simulink model "Testbed_OpenLoop"  (R2024b)
settings: Solver=VariableStepAuto  StartTime=0.0  StopTime=tf  RelTol=1e-3
values from neighbouring files (symbols this model uses):
  gamma1_initial = deg2rad(0)    [CMG_Testbed_Attitude_Control.m]
  gamma2_initial = deg2rad(0)    [CMG_Testbed_Attitude_Control.m]
libraries: simulink_extras x3, cstblocks x1
settings Model: Creator=lanhi  LastModifiedBy=lanhi

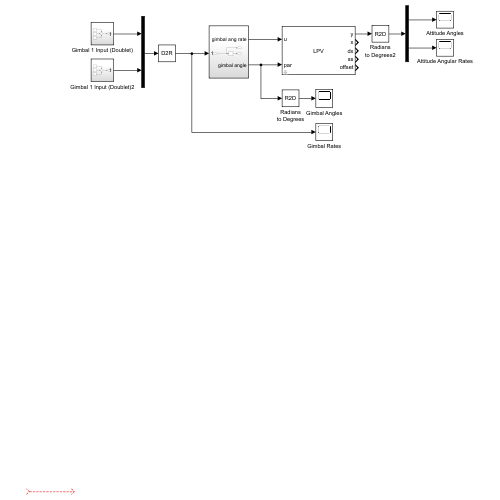
[thumbnail: Simulink's stored preview of the top-level diagram]
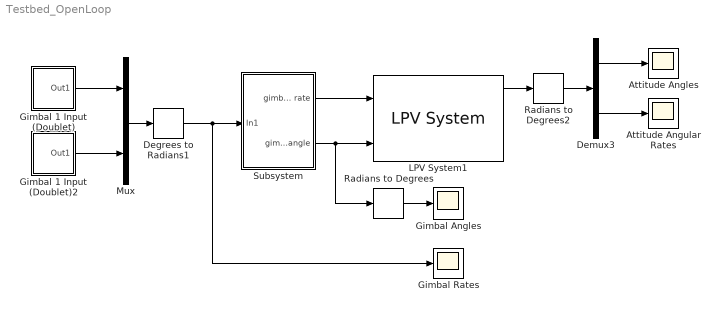
== system Testbed_OpenLoop ==
  Attitude Angles : Scope
  Attitude Angular Rates : Scope
  Degrees to Radians1 : simulink_extras/Transformations/Degrees to Radians
  Demux3 : Demux  Outputs=2
  Gimbal 1 Input (Doublet) : Subsystem
  Gimbal 1 Input (Doublet)2 : Subsystem
  Gimbal Angles : Scope
  Gimbal Rates : Scope
  LPV System1 : cstblocks/Linear Parameter Varying/LPV System  sys=ICs  InitialConditionSource=internal  InitialCondition=[deg2rad(0),0]  opSpecOption=Specify offsets as double arrays  uOffset=0  yOffset=0  xOffset=0  opEquilOption=on  dxOffset=0  AFixed=false  BFixed=false  CFixed=false  DFixed=false  uDelayFixed=false  yDelayFixed=false  iDelayFixed=false  sysFixedOption=First model in state-space array  sysFixed=[]  IMethod=Linear  EMethod=Clip  IndexSearch=Binary search  IndexBegin=on  OutputX=on  OutputXdot=on  OutputLTI=on  OutputOP=on  DataType=double  InitBufferSize=1024  FixedBuffer=off  SimMode=Interpreted execution  Offset=struct
  Mux : Mux  Inputs=2
  Radians to Degrees : simulink_extras/Transformations/Radians to Degrees
  Radians to Degrees2 : simulink_extras/Transformations/Radians to Degrees
  Subsystem : Subsystem
  wires:
  ? -> ?
  Radians to Degrees/1 -> Gimbal Angles/1
  Demux3/1 -> Attitude Angles/1
  Subsystem/2(gimbal angle) -> LPV System1/2, Radians to Degrees/1
  LPV System1/1 -> Radians to Degrees2/1
  Mux/1 -> Degrees to Radians1/1
  Subsystem/1(gimbal ang rate) -> LPV System1/1
  Radians to Degrees2/1 -> Demux3/1
  Demux3/2 -> Attitude Angular Rates/1
  Degrees to Radians1/1 -> Gimbal Rates/1, Subsystem/1(In1)
  Gimbal 1 Input (Doublet)/1(Out1) -> Mux/1
  Gimbal 1 Input (Doublet)2/1(Out1) -> Mux/2

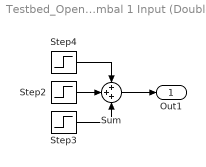
== system Testbed_OpenLoop/Gimbal 1 Input (Doublet) ==
  Step2 : Step  Time=5  After=-1  SampleTime=0
  Step3 : Step  Time=9  After=0.5  SampleTime=0
  Step4 : Step  After=0.5  SampleTime=0
  Sum : Sum  Inputs=+++
  Out1 : Outport
  wires:
  Step2/1 -> Sum/2
  Step4/1 -> Sum/1
  Step3/1 -> Sum/3
  Sum/1 -> Out1/1

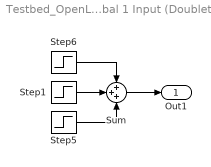
== system Testbed_OpenLoop/Gimbal 1 Input (Doublet)2 ==
  Step1 : Step  Time=5  After=-1  SampleTime=0
  Step5 : Step  Time=9  After=0.5  SampleTime=0
  Step6 : Step  After=0.5  SampleTime=0
  Sum : Sum  Inputs=+++
  Out1 : Outport
  wires:
  Step1/1 -> Sum/2
  Step6/1 -> Sum/1
  Step5/1 -> Sum/3
  Sum/1 -> Out1/1

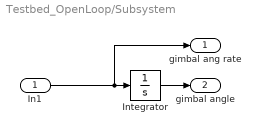
== system Testbed_OpenLoop/Subsystem ==
  In1 : Inport
  Integrator : Integrator  InitialCondition=[gamma1_initial,gamma2_initial]
  gimbal ang rate : Outport
  gimbal angle : Outport  Port=2
  wires:
  Integrator/1 -> gimbal angle/1
  In1/1 -> gimbal ang rate/1, Integrator/1
